simulink model "mjerenje_napona"  (R2015b)
settings: Solver=FixedStepAuto  StartTime=0.0  StopTime=inf  FixedStep=0.001  RelTol=1e-3
undefined symbols (not defined in the file): analoginput
libraries: daqlib x1
settings Model: Creator=ASIJA  LastModifiedBy=ASIJA

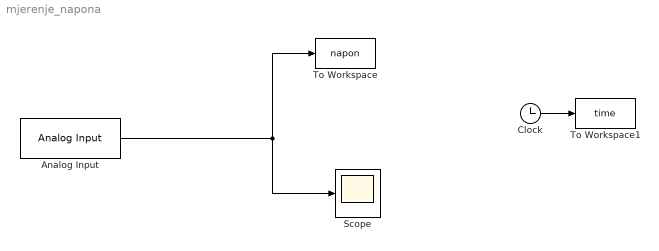
== system mjerenje_napona ==
  Analog Input : daqlib/Analog Input  AcqMode=0  DeviceMenu=mcc 1 (USB-1208FS)  Device=mcc 1 (USB-1208FS)  ObjConstructor=analoginput('mcc',1)  SampleRate=1000  ActualRate=1000  SamplesPerFrame=1  InputType=Differential  NChannelsSelected=1  Channels=0$0$$8$#0$1$$8$#1$2$$6$#0$3$$8$#  NPorts=1 for all hardware channels  DataType=double
      settings: SignalType=Sample-based
  Clock : Clock
  Scope : Scope
  To Workspace : ToWorkspace  VariableName=napon  SampleTime=-1
      settings: Save2DSignal=2-D array (concatenate along first dimension)
  To Workspace1 : ToWorkspace  VariableName=time  SampleTime=-1
  wires:
  Analog Input/1 -> To Workspace/1, Scope/1
  Clock/1 -> To Workspace1/1
